simulink model "model"  (R2019a)
settings: Solver=VariableStepAuto  StartTime=0.0  StopTime=840  RelTol=1e-3
values from neighbouring files (symbols this model uses):
  Q = 31.2    [workspace.mat]
undefined symbols (not defined in the file or in its folder): ocv, sigbuilder_block, soc
settings Model: Creator=sujan  LastModifiedBy=sujan

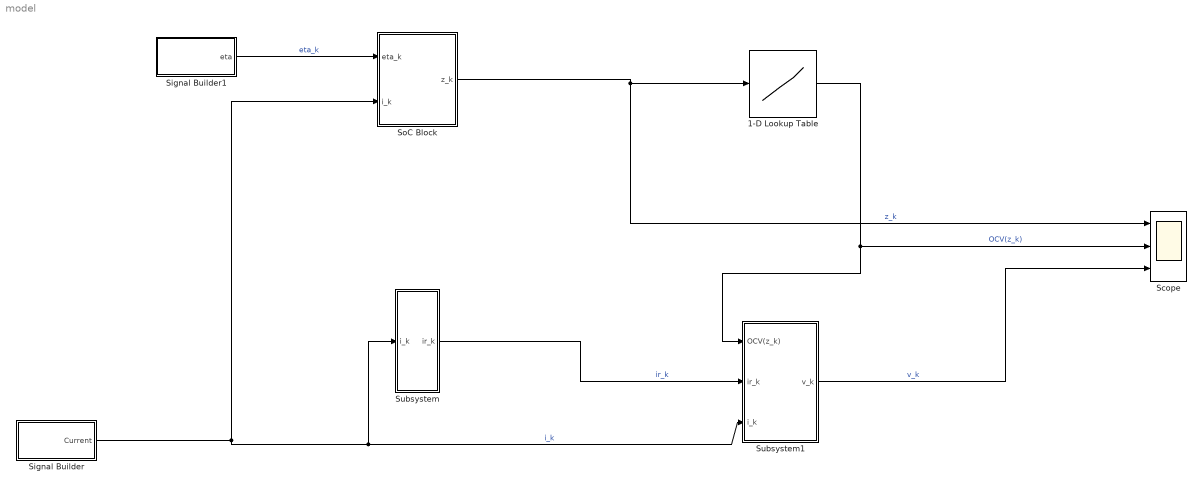
== system model ==
  1-D Lookup Table : Lookup_n-D  NumberOfTableDimensions=1  LookupTableObject=Em  BreakpointsForDimension1=soc.soc  Table=ocv.ocv  InternalRulePriority=Speed  RndMeth=Simplest  InputSameDT=on
  Scope : Scope  NumInputPorts=3
  Signal Builder : Subsystem  Tag=STV Subsys  LoadFcn=sigbuilder_block('load');  StartFcn=sigbuilder_block('start');  StopFcn=sigbuilder_block('stop');  ClipboardFcn=sigbuilder_block('clipboard');  mask(Sigbuilder block){tuvar=[0:10]}
      mask help: Simulink:masks:SigbuilderBlock_MD
      mask init:
      | if ~strcmp(get_param(bdroot(gcbh),'SimulationStatus'),'stopped') tuvar = sigbuilder_block('maskInit'); end
      settings: CopyFcn=sigbuilder_block('copy');  DeleteFcn=sigbuilder_block('delete');  ModelCloseFcn=sigbuilder_block('modelClose');  PreSaveFcn=sigbuilder_block('preSave');  PauseFcn=sigbuilder_block('pause');  ContinueFcn=sigbuilder_block('continue');  NameChangeFcn=sigbuilder_block('namechange');  OpenFcn=sigbuilder_block('open',[430.2 182.4 550.8 400.2 ]);  CloseFcn=sigbuilder_block('close');
      mask Display: plot(0, 0, 100, 100,[2, 2, 32, 32, 2], [68, 8, 8, 68, 68],[32, 2], [38, 38], [32, 19, 2],[53, 60, 44], [32, 17, 17, 2],[16, 16, 31, 31]);txt = getActiveGroup(gcbh);text(2, 100, txt,'verticalAlignment', 'top');
  Signal Builder1 : Subsystem  Tag=STV Subsys  LoadFcn=sigbuilder_block('load');  StartFcn=sigbuilder_block('start');  StopFcn=sigbuilder_block('stop');  ClipboardFcn=sigbuilder_block('clipboard');  mask(Sigbuilder block){tuvar=[0:10]}
      mask help: Simulink:masks:SigbuilderBlock_MD
      mask init:
      | if ~strcmp(get_param(bdroot(gcbh),'SimulationStatus'),'stopped') tuvar = sigbuilder_block('maskInit'); end
      settings: CopyFcn=sigbuilder_block('copy');  DeleteFcn=sigbuilder_block('delete');  ModelCloseFcn=sigbuilder_block('modelClose');  PreSaveFcn=sigbuilder_block('preSave');  PauseFcn=sigbuilder_block('pause');  ContinueFcn=sigbuilder_block('continue');  NameChangeFcn=sigbuilder_block('namechange');  OpenFcn=sigbuilder_block('open',[402.6 159.6 550.8 400.2 ]);  CloseFcn=sigbuilder_block('close');
      mask Display: plot(0, 0, 100, 100,[2, 2, 32, 32, 2], [68, 8, 8, 68, 68],[32, 2], [38, 38], [32, 19, 2],[53, 60, 44], [32, 17, 17, 2],[16, 16, 31, 31]);txt = getActiveGroup(gcbh);text(2, 100, txt,'verticalAlignment', 'top');
  "SoC Block " : Subsystem
  Subsystem : Subsystem
  Subsystem1 : Subsystem
  wires:
  1-D Lookup Table/1 -> Subsystem1/1(OCV(z_k)), Scope/2  "OCV(z_k)"
  Signal Builder/1(Current) -> Subsystem/1(i_k), Subsystem1/3(i_k), "SoC Block "/2(i_k)  "i_k"
  "SoC Block "/1(z_k) -> Scope/1, 1-D Lookup Table/1  "z_k"
  Signal Builder1/1(eta) -> "SoC Block "/1(eta_k)  "eta_k"
  Subsystem/1(ir_k) -> Subsystem1/2(ir_k)  "ir_k"
  Subsystem1/1(v_k) -> Scope/3  "v_k"

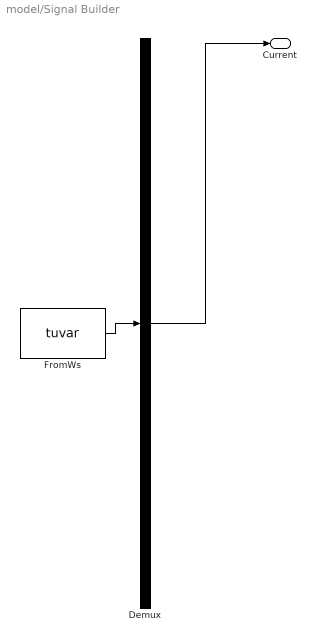
== system model/Signal Builder ==
  Demux : Demux  Tag=STV Demux  Outputs=1
  FromWs : FromWorkspace  Tag=STV FromWs  VariableName=tuvar  SampleTime=0
      SigBuilderData=|
      | common.afterFinalStr = 'Extrapolate'
      | common.sampleTime = 0
      | dataSet.timeRange = [0.014126552 106.3976602]
      | dataSet.name = 'svsd'
      | sbobj.Groups.Name = 'svsd'
      | sbobj.Groups.Signals.Name = 'Current'
      | sbobj.Groups.Signals.XData = [0.014126552 0.114126552 0.217169883 0.304839902 0.382614986 0.453299094 0.518566067 0.579514007 0.636910647 0.691318351 0.743164033 0.79278106 ... (9908 elements, 1x9908)]
      | sbobj.Groups.Signals.YData = [12.71758197 11.90678231 11.9322143 11.95390158 11.97317805 11.98962184 12.00453334 12.01847546 12.03162035 12.0440941 12.05599245 12.06739015 ... (9908 elements, 1x9908)]
      | sbobj.Groups.TimeRange = [0.014126552 106.3976602]
  Current : Outport  Tag=STV Outport
  wires:
  Demux/1 -> Current/1
  FromWs/1 -> Demux/1

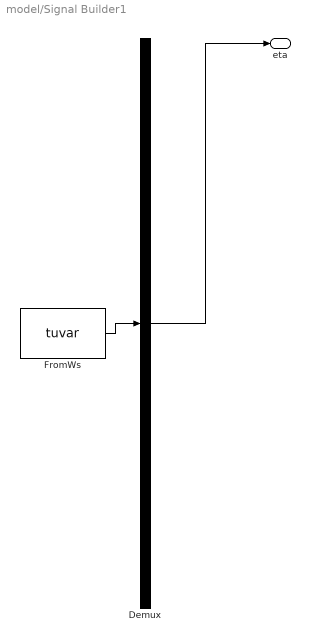
== system model/Signal Builder1 ==
  Demux : Demux  Tag=STV Demux  Outputs=1
  FromWs : FromWorkspace  Tag=STV FromWs  VariableName=tuvar  SampleTime=0
      SigBuilderData=|
      | common.afterFinalStr = 'Extrapolate'
      | common.sampleTime = 0
      | dataSet.timeRange = [0.014126552 106.3976602]
      | dataSet.name = 'svsd'
      | sbobj.Groups.Name = 'svsd'
      | sbobj.Groups.Signals.Name = 'eta'
      | sbobj.Groups.Signals.XData = [0.014126552 0.114126552 0.217169883 0.304839902 0.382614986 0.453299094 0.518566067 0.579514007 0.636910647 0.691318351 0.743164033 0.79278106 ... (9908 elements, 1x9908)]
      | sbobj.Groups.Signals.YData = [0.96345318 0.902028963 0.903955629 0.905598605 0.907058943 0.908304685 0.909434344 0.910490565 0.91148639 0.912431371 0.913332761 0.914196223 ... (9908 elements, 1x9908)]
  eta : Outport  Tag=STV Outport
  wires:
  Demux/1 -> eta/1
  FromWs/1 -> Demux/1

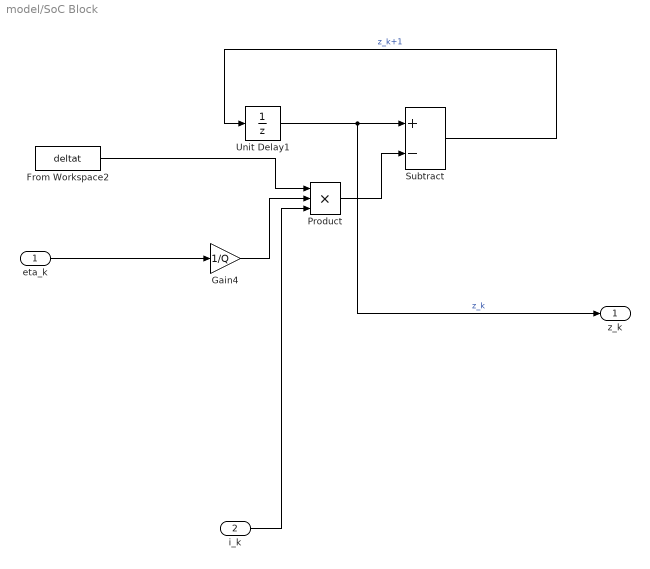
== system model/SoC Block  ==
  eta_k : Inport
  i_k : Inport  Port=2
  From Workspace2 : FromWorkspace  VariableName=deltat  SampleTime=0
  Gain4 : Gain  Gain=1/Q
  Product : Product  Inputs=3
  Subtract : Sum  Inputs=+-
  Unit Delay1 : UnitDelay  InitialCondition=100  HasFrameUpgradeWarning=on
  z_k : Outport
  wires:
  Product/1 -> Subtract/2
  From Workspace2/1 -> Product/1
  Unit Delay1/1 -> z_k/1, Subtract/1  "z_k"
  eta_k/1 -> Gain4/1
  Gain4/1 -> Product/2
  i_k/1 -> Product/3
  Subtract/1 -> Unit Delay1/1  "z_k+1"

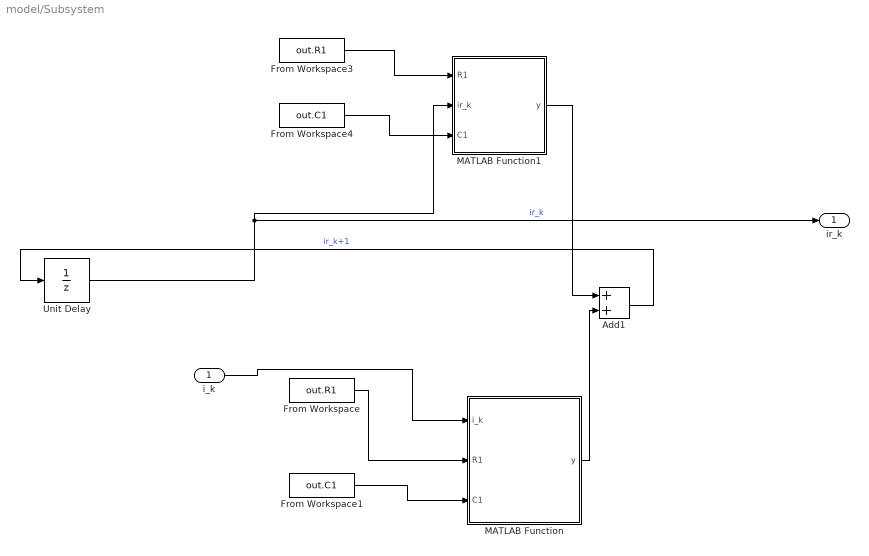
== system model/Subsystem ==
  i_k : Inport
  Add1 : Sum
  From Workspace : FromWorkspace  VariableName=out.R1  SampleTime=0
  From Workspace1 : FromWorkspace  VariableName=out.C1  SampleTime=0
  From Workspace3 : FromWorkspace  VariableName=out.R1  SampleTime=0
  From Workspace4 : FromWorkspace  VariableName=out.C1  SampleTime=0
  MATLAB Function : MATLAB Function  TreatAsAtomicUnit=on
  MATLAB Function1 : MATLAB Function  TreatAsAtomicUnit=on
  Unit Delay : UnitDelay  SampleTime=0.5  HasFrameUpgradeWarning=on
  ir_k : Outport
  wires:
  MATLAB Function1/1(y) -> Add1/1
  Unit Delay/1 -> MATLAB Function1/2(ir_k), ir_k/1  "ir_k"
  Add1/1 -> Unit Delay/1  "ir_k+1"
  i_k/1 -> MATLAB Function/1(i_k)
  MATLAB Function/1(y) -> Add1/2
  From Workspace/1 -> MATLAB Function/2(R1)
  From Workspace4/1 -> MATLAB Function1/3(C1)
  From Workspace3/1 -> MATLAB Function1/1(R1)
  From Workspace1/1 -> MATLAB Function/3(C1)

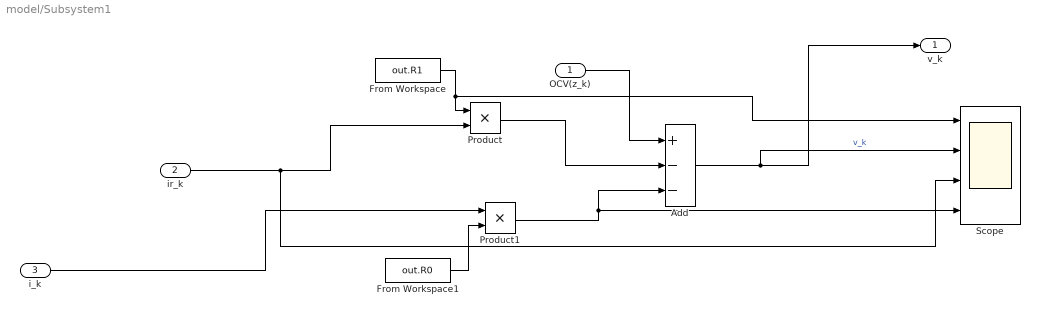
== system model/Subsystem1 ==
  OCV(z_k) : Inport
  ir_k : Inport  Port=2
  i_k : Inport  Port=3
  Add : Sum  Inputs=+--
  From Workspace : FromWorkspace  VariableName=out.R1  SampleTime=0
  From Workspace1 : FromWorkspace  VariableName=out.R0  SampleTime=0
  Product : Product
  Product1 : Product
  Scope : Scope  NumInputPorts=4
  v_k : Outport
  wires:
  ir_k/1 -> Scope/3, Product/2
  Product/1 -> Add/2
  Product1/1 -> Scope/4, Add/3
  i_k/1 -> Product1/1
  OCV(z_k)/1 -> Add/1
  Add/1 -> Scope/2, v_k/1  "v_k"
  From Workspace1/1 -> Product1/2
  From Workspace/1 -> Scope/1, Product/1

== matlab function model/Subsystem/MATLAB Function1 ==
  data: R1 input; ir_k input; C1 input; y output
function y = fcn(R1,ir_k, C1)
deltat = 0.010737239;
y =ir_k*(exp(-deltat/(R1*C1)));

== matlab function model/Subsystem/MATLAB Function ==
  data: i_k input; R1 input; C1 input; y output
function y = fcn(i_k, R1,C1)
deltat= 0.010737239;
y = i_k*(1-exp(-deltat/(R1*C1)));
